simulink model "sampleModel1723"  (R2023a)
settings: Solver=VariableStepAuto  StartTime=0.0  StopTime=10.0  RelTol=1e-3
libraries: hdlsllib x7
settings Model: Creator=user1  LastModifiedBy=user1

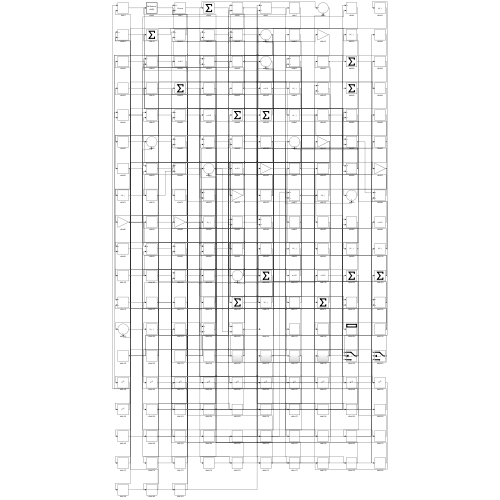
[thumbnail: Simulink's stored preview of the top-level diagram]
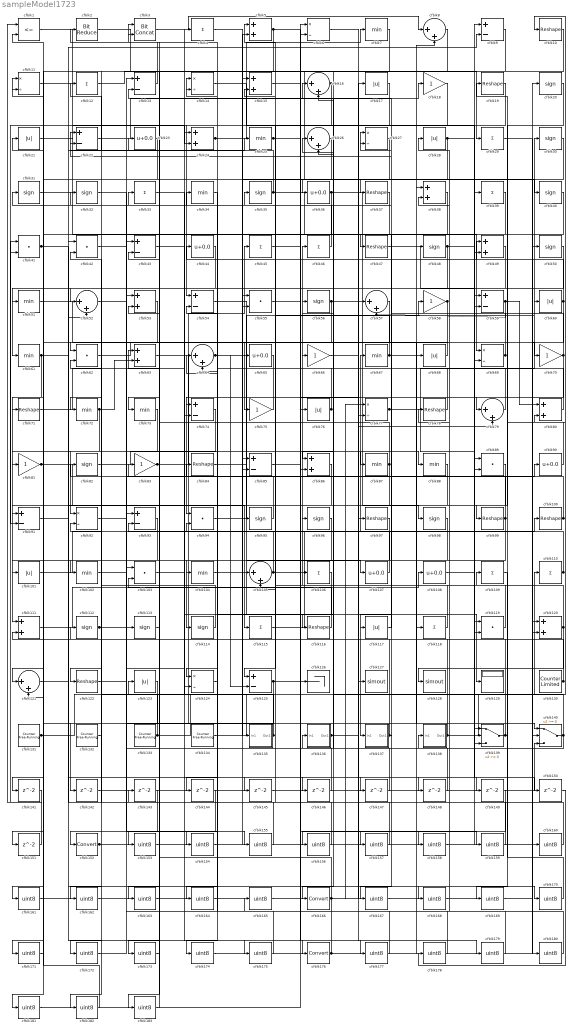
== system sampleModel1723 ==
  cfblk1 : RelationalOperator  Operator=<=  OutDataTypeStr=boolean  InputSameDT=off
  cfblk{10,19,37,47,71,78,84,97,99..100,116,122} (12 alike) : Reshape
  cfblk{17,21,28,60,68,76,101,117,123} (9 alike) : Abs  SaturateOnIntegerOverflow=off
  cfblk{7,25,34,51,61,67,72..73,87..88,102,104} (12 alike) : MinMax
  cfblk{41..42,55,62,89,94,103,119} (8 alike) : DotProduct  OutDataTypeStr=Inherit: Inherit via internal rule
  cfblk{8,16,26,52,57,64,79,105,121} (9 alike) : Sum  Inputs=|++
  cfblk{4,12,29,33,39,45..46,106,109..110,115,118} (12 alike) : Sum  Inputs=+
  cfblk{23,36,44,65,90,107..108} (7 alike) : Bias  Bias=0.0  SaturateOnIntegerOverflow=off
  cfblk{6,11,14,27,69,77,92,124} (8 alike) : Product  Inputs=*/  RndMeth=Zero  SaturateOnIntegerOverflow=on
  cfblk{5,15,24,38,49,53,63,80,86,111,120} (11 alike) : Sum
  cfblk{20,30..32,35,40,48,50,56,82,95..96,98,112..114} (16 alike) : Signum
  cfblk{9,13,22,43,54,59,74,85,91,93,125} (11 alike) : Sum  Inputs=+-
  cfblk126 : Terminator
  cfblk127 : ToWorkspace  VariableName=simout  SaveFormat=Timeseries  SampleTime=-1
  cfblk128 : ToWorkspace  VariableName=simout  SaveFormat=Timeseries  SampleTime=-1
  cfblk129 : Display
  cfblk130 : hdlsllib/Sources/Counter Limited  uplimit=7  tsamp=-1
  cfblk{131..134} (4 alike) : hdlsllib/Sources/Counter Free-Running  NumBits=16  tsamp=-1
  cfblk135 : Subsystem
      settings: LibrarySourceBlock=|
      | hdlsllib/Ports &
      | Subsystems/Subsystem
  cfblk136 : Subsystem
      settings: LibrarySourceBlock=|
      | hdlsllib/Ports &
      | Subsystems/Subsystem
  cfblk137 : Subsystem
      settings: LibrarySourceBlock=|
      | hdlsllib/Ports &
      | Subsystems/Subsystem
  cfblk138 : Subsystem
      settings: LibrarySourceBlock=|
      | hdlsllib/Ports &
      | Subsystems/Subsystem
  cfblk139 : Switch  SaturateOnIntegerOverflow=off  InputSameDT=off
  cfblk140 : Switch  SaturateOnIntegerOverflow=off  InputSameDT=off
  cfblk{141..151} (11 alike) : Delay  SampleTime=1
  cfblk152 : DataTypeConversion  SaturateOnIntegerOverflow=off  RndMeth=Floor
  cfblk{153..165,167..175,177..183} (29 alike) : DataTypeConversion  OutDataTypeStr=uint8  SaturateOnIntegerOverflow=off  RndMeth=Floor
  cfblk166 : DataTypeConversion  SaturateOnIntegerOverflow=off  RndMeth=Floor
  cfblk176 : DataTypeConversion  SaturateOnIntegerOverflow=off  RndMeth=Floor
  cfblk{18,58,66,70,75,81,83} (7 alike) : Gain
  cfblk2 : hdlsllib/Logic and Bit Operations/Bit Reduce  mode=AND
  cfblk3 : hdlsllib/Logic and Bit Operations/Bit Concat  numInputs=2
  wires:
  cfblk3/1 -> cfblk8/1
  cfblk77/1 -> cfblk30/1, cfblk119/1
  cfblk112/1 -> cfblk113/1, cfblk139/2
  cfblk36/1 -> cfblk98/1, cfblk74/2
  cfblk25/1 -> cfblk159/1, cfblk177/1
  cfblk120/1 -> cfblk46/1, cfblk84/1, cfblk128/1
  cfblk12/1 -> cfblk37/1
  cfblk88/1 -> cfblk115/1
  cfblk10/1 -> cfblk86/1
  cfblk16/1 -> cfblk54/1, cfblk105/2
  cfblk2/1 -> cfblk29/1
  cfblk140/1 -> cfblk136/1(In1), cfblk96/1
  cfblk130/1 -> cfblk56/1, cfblk11/1
  cfblk118/1 -> cfblk16/1
  cfblk110/1 -> cfblk67/1, cfblk28/1
  cfblk125/1 -> cfblk126/1, cfblk142/1
  cfblk117/1 -> cfblk27/1
  cfblk21/1 -> cfblk47/1
  cfblk78/1 -> cfblk26/1
  cfblk61/1 -> cfblk111/1, cfblk145/1
  cfblk99/1 -> cfblk27/2, cfblk114/1
  cfblk83/1 -> cfblk45/1, cfblk119/2
  cfblk68/1 -> cfblk62/1
  cfblk94/1 -> cfblk58/1
  cfblk138/1(Out1) -> cfblk10/1, cfblk111/2, cfblk11/2, cfblk78/1
  cfblk38/1 -> cfblk166/1
  cfblk44/1 -> cfblk61/1
  cfblk100/1 -> cfblk3/1, cfblk80/2
  cfblk131/1 -> cfblk24/1, cfblk9/1
  cfblk45/1 -> cfblk77/2
  cfblk84/1 -> cfblk137/1(In1)
  cfblk62/1 -> cfblk70/1
  cfblk48/1 -> cfblk150/1, cfblk157/1
  cfblk72/1 -> cfblk81/1, cfblk63/2
  cfblk73/1 -> cfblk92/1
  cfblk85/1 -> cfblk60/1
  cfblk27/1 -> cfblk73/1
  cfblk35/1 -> cfblk69/1, cfblk12/1
  cfblk24/1 -> cfblk7/1, cfblk40/1
  cfblk107/1 -> cfblk33/1
  cfblk5/1 -> cfblk76/1, cfblk52/1
  cfblk69/1 -> cfblk13/2, cfblk22/2
  cfblk18/1 -> cfblk122/1
  cfblk63/1 -> cfblk140/1
  cfblk111/1 -> cfblk108/1
  cfblk9/1 -> cfblk86/2
  cfblk65/1 -> cfblk94/1
  cfblk70/1 -> cfblk124/1, cfblk79/1, cfblk32/1
  cfblk115/1 -> cfblk100/1
  cfblk101/1 -> cfblk57/1
  cfblk23/1 -> cfblk121/1
  cfblk60/1 -> cfblk19/1, cfblk120/2
  cfblk139/1 -> cfblk49/1, cfblk63/1
  cfblk67/1 -> cfblk5/1, cfblk139/3
  cfblk41/1 -> cfblk25/1, cfblk95/1
  cfblk74/1 -> cfblk91/1
  cfblk132/1 -> cfblk112/1
  cfblk11/1 -> cfblk59/1
  cfblk32/1 -> cfblk124/2
  cfblk31/1 -> cfblk59/2
  cfblk97/1 -> cfblk125/1
  cfblk59/1 -> cfblk57/2, cfblk80/1
  cfblk114/1 -> cfblk62/2
  cfblk19/1 -> cfblk91/2
  cfblk86/1 -> cfblk121/2
  cfblk136/1(Out1) -> cfblk97/1, cfblk168/1
  cfblk64/1 -> cfblk107/1, cfblk125/2
  cfblk79/1 -> cfblk22/1
  cfblk54/1 -> cfblk129/1
  cfblk124/1 -> cfblk64/2
  cfblk56/1 -> cfblk75/1, cfblk116/1, cfblk79/2
  cfblk108/1 -> cfblk49/2
  cfblk105/1 -> cfblk101/1, cfblk14/1, cfblk48/1
  cfblk119/1 -> cfblk66/1
  cfblk37/1 -> cfblk71/1
  cfblk47/1 -> cfblk139/1
  cfblk116/1 -> cfblk103/2
  cfblk26/1 -> cfblk36/1
  cfblk22/1 -> cfblk18/1
  cfblk55/1 -> cfblk88/1
  cfblk104/1 -> cfblk5/2
  cfblk71/1 -> cfblk4/1
  cfblk137/1(Out1) -> cfblk54/2, cfblk167/1
  cfblk87/1 -> cfblk23/1, cfblk104/1
  cfblk8/1 -> cfblk51/1
  cfblk14/1 -> cfblk69/2
  cfblk90/1 -> cfblk44/1
  cfblk89/1 -> cfblk152/1
  cfblk66/1 -> cfblk127/1
  cfblk134/1 -> cfblk110/1
  cfblk133/1 -> cfblk55/2, cfblk85/1, cfblk123/1
  cfblk81/1 -> cfblk135/1(In1), cfblk52/2, cfblk9/2
  cfblk51/1 -> cfblk118/1
  cfblk20/1 -> cfblk99/1
  cfblk17/1 -> cfblk41/2
  cfblk82/1 -> cfblk87/1
  cfblk46/1 -> cfblk31/1
  cfblk39/1 -> cfblk117/1
  cfblk28/1 -> cfblk39/1, cfblk72/1
  cfblk4/1 -> cfblk105/1
  cfblk80/1 -> cfblk26/2
  cfblk135/1(Out1) -> cfblk92/2, cfblk35/1
  cfblk52/1 -> cfblk65/1
  cfblk43/1 -> cfblk176/1
  cfblk92/1 -> cfblk90/1
  cfblk96/1 -> cfblk102/1
  cfblk58/1 -> cfblk85/2, cfblk154/1
  cfblk75/1 -> cfblk74/1
  cfblk76/1 -> cfblk3/2, cfblk14/2
  cfblk95/1 -> cfblk82/1
  cfblk1/1 -> cfblk24/2
  cfblk13/1 -> cfblk2/1
  cfblk57/1 -> cfblk141/1
  cfblk141/1 -> cfblk1/1
  cfblk142/1 -> cfblk8/2
  cfblk49/1 -> cfblk144/1
  cfblk145/1 -> cfblk140/3
  cfblk33/1 -> cfblk146/1
  cfblk146/1 -> cfblk64/1
  cfblk122/1 -> cfblk147/1
  cfblk147/1 -> cfblk13/1
  cfblk102/1 -> cfblk148/1
  cfblk148/1 -> cfblk16/2
  cfblk103/1 -> cfblk149/1
  cfblk50/1 -> cfblk151/1
  cfblk151/1 -> cfblk41/1
  cfblk152/1 -> cfblk120/1, cfblk55/1
  cfblk113/1 -> cfblk153/1
  cfblk153/1 -> cfblk89/1
  cfblk154/1 -> cfblk89/2
  cfblk42/1 -> cfblk155/1
  cfblk155/1 -> cfblk103/1
  cfblk149/1 -> cfblk156/1
  cfblk156/1 -> cfblk42/1
  cfblk157/1 -> cfblk42/2
  cfblk15/1 -> cfblk158/1
  cfblk158/1 -> cfblk50/1
  cfblk159/1 -> cfblk15/1
  cfblk160/1 -> cfblk15/2
  cfblk53/1 -> cfblk161/1
  cfblk161/1 -> cfblk17/1
  cfblk144/1 -> cfblk162/1
  cfblk162/1 -> cfblk53/1
  cfblk7/1 -> cfblk163/1
  cfblk163/1 -> cfblk53/2
  cfblk106/1 -> cfblk164/1
  cfblk164/1 -> cfblk20/1
  cfblk165/1 -> cfblk106/1
  cfblk166/1 -> cfblk165/1, cfblk83/1, cfblk77/1
  cfblk167/1 -> cfblk38/1
  cfblk168/1 -> cfblk38/2
  cfblk109/1 -> cfblk169/1
  cfblk169/1 -> cfblk140/2
  cfblk121/1 -> cfblk170/1
  cfblk170/1 -> cfblk109/1
  cfblk93/1 -> cfblk171/1
  cfblk171/1 -> cfblk21/1
  cfblk98/1 -> cfblk172/1
  cfblk172/1 -> cfblk93/1
  cfblk40/1 -> cfblk173/1
  cfblk173/1 -> cfblk93/2
  cfblk34/1 -> cfblk174/1
  cfblk174/1 -> cfblk68/1
  cfblk91/1 -> cfblk175/1
  cfblk175/1 -> cfblk34/1
  cfblk176/1 -> cfblk160/1, cfblk94/2
  cfblk177/1 -> cfblk43/1
  cfblk150/1 -> cfblk178/1
  cfblk178/1 -> cfblk43/2
  cfblk6/1 -> cfblk179/1
  cfblk179/1 -> cfblk138/1(In1)
  cfblk29/1 -> cfblk180/1
  cfblk180/1 -> cfblk6/1
  cfblk123/1 -> cfblk181/1
  cfblk181/1 -> cfblk6/2
  cfblk143/1 -> cfblk182/1
  cfblk182/1 -> cfblk1/2
  cfblk30/1 -> cfblk183/1
  cfblk183/1 -> cfblk143/1

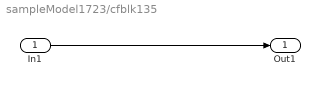
== system sampleModel1723/cfblk135 ==
  In1 : Inport
  Out1 : Outport
  wires:
  In1/1 -> Out1/1

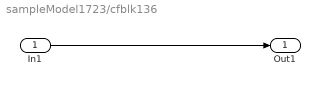
== system sampleModel1723/cfblk136 ==
  In1 : Inport
  Out1 : Outport
  wires:
  In1/1 -> Out1/1

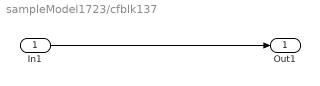
== system sampleModel1723/cfblk137 ==
  In1 : Inport
  Out1 : Outport
  wires:
  In1/1 -> Out1/1

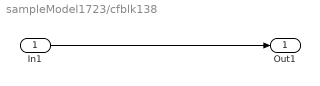
== system sampleModel1723/cfblk138 ==
  In1 : Inport
  Out1 : Outport
  wires:
  In1/1 -> Out1/1
